simulink model "LedResponseToZAcceleration"  (R2013b)
settings: Solver=FixedStepDiscrete  StartTime=0.0  StopTime=60  FixedStep=0.1  RelTol=1e-3
libraries: ardrone_lib x2, simulink x2
settings Model: Creator=Jon Even ROSENGREN  LastModifiedBy=Jon Even ROSENGREN
settings DataIOCC: SignalLoggingSaveFormat=ModelDataLogs
settings OptimizationCC: InitFltsAndDblsToZero=on  OptimizeModelRefInitCode=on  LifeSpan=1
settings DebuggingCC: MultiTaskDSMMsg=warning  MultiTaskCondExecSysMsg=none  StrictBusMsg=None
settings RTWCC: SystemTargetFile=ardrone.tlc  TemplateMakefile=ardrone.tmf  Description=AR.Drone_v2  ProcessScript=ardrone_make_rtw_hook  TargetLang=C++  IncludeERTFirstTime=on
settings CodeAppCC: IgnoreCustomStorageClasses=off
settings STFCustomTargetCC: GenerateSampleERTMain=on  ModelReferenceCompliant=off  CombineOutputUpdateFcns=on  ERTCustomFileBanners=on  SupportContinuousTime=off  SupportNonInlinedSFcns=off  MATLABClassNameForMDSCustomization=Simulink.SoftwareTarget.ERTCustomization  GRTInterface=off  SystemTargetFile=ardrone.tlc
settings ERTTargetCC: CodeReplacementLibrary=ANSI_C  GenerateSampleERTMain=on  ModelReferenceCompliant=off  ParMdlRefBuildCompliant=off  CompOptLevelCompliant=off  ConcurrentExecutionCompliant=off  ERTFirstTimeCompliant=off  ModelStepFunctionPrototypeControlCompliant=off  CPPClassGenCompliant=off  ERTSrcFileBannerTemplate=example_banner.tlc  ERTHdrFileBannerTemplate=example_banner.tlc  ERTCustomFileTemplate=ardrone_file_process.tlc

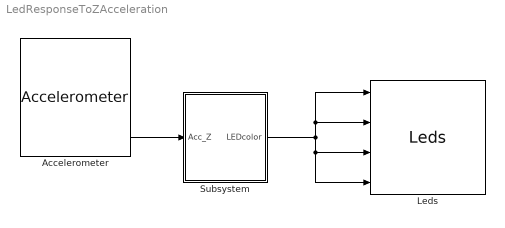
== system LedResponseToZAcceleration ==
  Accelerometer : ardrone_lib/Accelerometer  SystemSampleTime=-1
  Leds : ardrone_lib/Leds  SystemSampleTime=-1
  Subsystem : Subsystem
  wires:
  Accelerometer/3 -> Subsystem/1(Acc_Z)
  Subsystem/1(LEDcolor) -> Leds/4, Leds/3, Leds/2, Leds/1

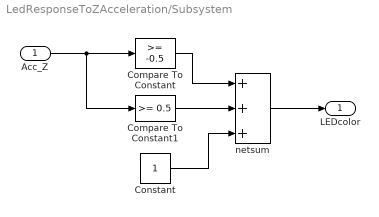
== system LedResponseToZAcceleration/Subsystem ==
  Acc_Z : Inport
  Compare To Constant : simulink/Logic and Bit Operations/Compare To Constant  relop=>=  const=-0.5  OutDataTypeStr=uint8
  Compare To Constant1 : simulink/Logic and Bit Operations/Compare To Constant  relop=>=  const=0.5  OutDataTypeStr=uint8
  Constant : Constant  OutDataTypeStr=uint8
  netsum : Sum  Inputs=+++  SaturateOnIntegerOverflow=on  InputSameDT=on  OutDataTypeStr=Inherit: Same as first input
  LEDcolor : Outport
  wires:
  Acc_Z/1 -> Compare To Constant1/1, Compare To Constant/1
  netsum/1 -> LEDcolor/1
  Compare To Constant/1 -> netsum/1
  Compare To Constant1/1 -> netsum/2
  Constant/1 -> netsum/3
